simulink model "HANcoder_E407_GTSync_v5"  (R2018b)
settings: Solver=FixedStepDiscrete  StartTime=0.0  StopTime=1  FixedStep=0.01  RelTol=1e-3
PreLoadFcn:
  | librarySetup
  | eval([bdroot,'_startup']) %Calling [modelName]_startup.m
values from neighbouring files (symbols this model uses):
  basic_cycle_duration = TM_Reset_Board + COMP_duration    (= 170)    [HANcoder_E407_GTSync_v5_startup.m]
  comm_delay_estimation1 = round(comm_delay_measured*hardware_granularity/frequency_IRQ)    [HANcoder_E407_GTSync_v5_startup.m]
  comm_delay_estimation2 = round(comm_delay_measured*hardware_granularity/frequency_IRQ)    [HANcoder_E407_GTSync_v5_startup.m]
  COMM_Period = 25    [HANcoder_E407_GTSync_v5_startup.m]
  COMM_Phase1 = floor(COMM_Period/5)    [HANcoder_E407_GTSync_v5_startup.m]
  COMM_Phase2 = floor(4*COMM_Period/5)    [HANcoder_E407_GTSync_v5_startup.m]
  frequency_IRQ = 100    [HANcoder_E407_GTSync_v5_startup.m]
  HANtuneOverride = Simulink.Parameter    [HANcoder_E407_GTSync_v5_startup.m]
  idle_time_init = basic_cycle_duration*matrix_rows    (= 340)    [HANcoder_E407_GTSync_v5_startup.m]
  LED_ticks_toggle = 10000    [HANcoder_E407_GTSync_v5_startup.m]
  Master_Role = 1    [HANcoder_E407_GTSync_v5_startup.m]
  matrix_rows = 2    [HANcoder_E407_GTSync_v5_startup.m]
  MEX_Flag = 0    [HANcoder_E407_GTSync_v5_startup.m]
  Slave_Role = 2    [HANcoder_E407_GTSync_v5_startup.m]
  Sync_ID = 1    [HANcoder_E407_GTSync_v5_startup.m]
  TM_Check_Sync = TM_COMM_Sync   + COMM_duration    (= 30)    [HANcoder_E407_GTSync_v5_startup.m]
  TM_Check_TOuts = TM_Count_Vote3 + COMP_duration    (= 150)    [HANcoder_E407_GTSync_v5_startup.m]
  TM_Check_Vote1 = TM_COMM_Vote1  + COMM_duration    (= 70)    [HANcoder_E407_GTSync_v5_startup.m]
  TM_Check_Vote2 = TM_COMM_Vote2  + COMM_duration    (= 105)    [HANcoder_E407_GTSync_v5_startup.m]
  TM_Check_Vote3 = TM_COMM_Vote3  + COMM_duration    (= 140)    [HANcoder_E407_GTSync_v5_startup.m]
  TM_COMM_Sync = basic_cycle_start    (= 5)    [HANcoder_E407_GTSync_v5_startup.m]
  TM_COMM_Vote1 = TM_Vote_Dec    + COMP_duration    (= 45)    [HANcoder_E407_GTSync_v5_startup.m]
  TM_COMM_Vote2 = TM_Count_Vote1 + COMP_duration    (= 80)    [HANcoder_E407_GTSync_v5_startup.m]
  TM_COMM_Vote3 = TM_Count_Vote2 + COMP_duration    (= 115)    [HANcoder_E407_GTSync_v5_startup.m]
  TM_Count_Vote1 = TM_Check_Vote1 + COMP_duration    (= 75)    [HANcoder_E407_GTSync_v5_startup.m]
  TM_Count_Vote2 = TM_Check_Vote2 + COMP_duration    (= 110)    [HANcoder_E407_GTSync_v5_startup.m]
  TM_Count_Vote3 = TM_Check_Vote3 + COMP_duration    (= 145)    [HANcoder_E407_GTSync_v5_startup.m]
  TM_New_Master = TM_Check_TOuts + COMP_duration    (= 155)    [HANcoder_E407_GTSync_v5_startup.m]
  TM_Reset_Board = TM_Reset_Var   + COMP_duration    (= 165)    [HANcoder_E407_GTSync_v5_startup.m]
  TM_Reset_Var = TM_New_Master  + COMP_duration    (= 160)    [HANcoder_E407_GTSync_v5_startup.m]
  TM_Update_LT = TM_Check_Sync  + COMP_duration    (= 35)    [HANcoder_E407_GTSync_v5_startup.m]
  TM_Vote_Dec = TM_Update_LT   + COMP_duration    (= 40)    [HANcoder_E407_GTSync_v5_startup.m]
  Toggle_Flag = 1    [HANcoder_E407_GTSync_v5_startup.m]
  Vote1_ID = 12    [HANcoder_E407_GTSync_v5_startup.m]
  Vote2_ID = 22    [HANcoder_E407_GTSync_v5_startup.m]
  Vote3_ID = 32    [HANcoder_E407_GTSync_v5_startup.m]
undefined symbols (not defined in the file or in its folder): A0, A1, A2, A3, CON2
libraries: HANcoder_STM32_Target x25, hdlsllib x21, simulink x3, simulink_extras x1
(part 3 of 7)

== system HANcoder_E407_GTSync_v5/HANcoder STM32 Target - E407-STM32 algorithm/Global Ticks Increment/CAN Management/Initialization/RoleID and Global Time init ==
  note: Sync msg received!
  note: Reset variables
  note: Finish Initialization
  note: Role_ID Initialization
  Timeout Initialization : Inport
  Reference message received : Inport  Port=2
  Enable : EnablePort
  Constant : Constant  Priority=4  Value=Master_Role
  Constant1 : Constant  Priority=3  Value=Slave_Role
  Data Store Read : DataStoreRead  Priority=5  DataStoreName=Role_ID
  Data Store Write : DataStoreWrite  Priority=8  DataStoreName=Role_ID
  Data Store Write1 : DataStoreWrite  Priority=10  DataStoreName=sync_processed
  Data Store Write2 : DataStoreWrite  Priority=18  DataStoreName=Delay_Counter
  Data Store Write3 : DataStoreWrite  Priority=12  DataStoreName=New_Msg_Ready_CAN1
  Data Store Write4 : DataStoreWrite  Priority=16  DataStoreName=Initialization_Timeout
  Data Store Write5 : DataStoreWrite  Priority=14  DataStoreName=New_Msg_Ready_CAN2
  Global Time Initialization Master : Subsystem  Priority=2
  Global Time Initialization Slave : Subsystem  Priority=1
  RESET : Constant  Priority=15  Value=0  OutDataTypeStr=boolean
  RESET1 : Constant  Priority=17  Value=0  OutDataTypeStr=double
  RESET2 : Constant  Priority=11  Value=0  OutDataTypeStr=boolean
  RESET3 : Constant  Priority=13  Value=0  OutDataTypeStr=boolean
  SET : Constant  Priority=19
  "SET1 " : Constant  Priority=9  OutDataTypeStr=boolean
  Switch1 : Switch  Priority=6  Criteria=u2 > Threshold
  Switch2 : Switch  Priority=7  Criteria=u2 > Threshold
  Finish Initialization : Outport  OutputWhenDisabled=reset  InitialOutput=0
  wires:
  Switch1/1 -> Switch2/3
  Reference message received/1 -> Global Time Initialization Slave/Enable, Switch2/2
  Data Store Read/1 -> Switch1/3
  SET/1 -> Finish Initialization/1
  Constant/1 -> Switch1/1
  Constant1/1 -> Switch2/1
  Switch2/1 -> Data Store Write/1
  RESET/1 -> Data Store Write4/1
  Timeout Initialization/1 -> Switch1/2, Global Time Initialization Master/Enable
  RESET1/1 -> Data Store Write2/1
  "SET1 "/1 -> Data Store Write1/1
  RESET2/1 -> Data Store Write3/1
  RESET3/1 -> Data Store Write5/1

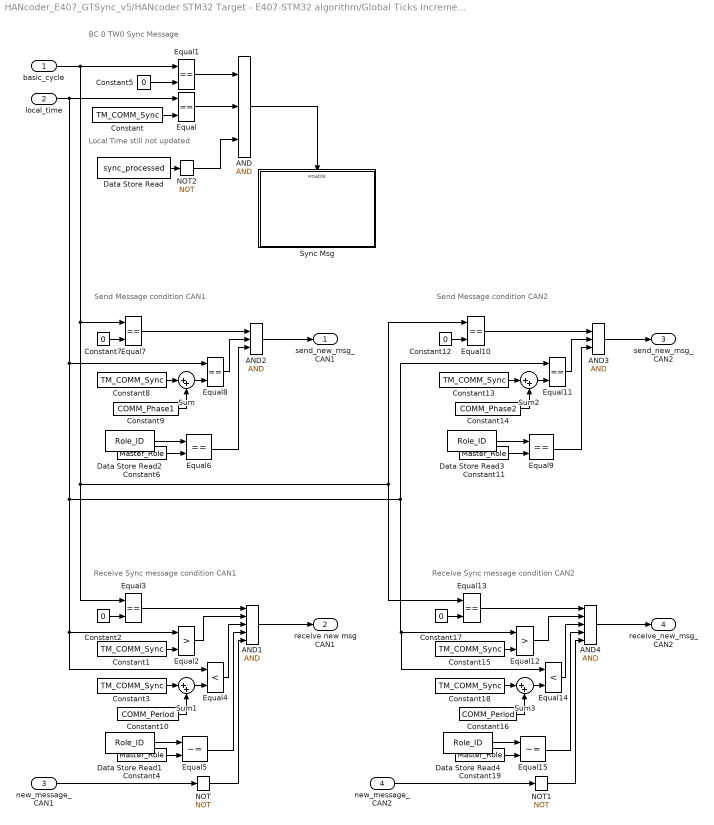
== system HANcoder_E407_GTSync_v5/HANcoder STM32 Target - E407-STM32 algorithm/Global Ticks Increment/CAN Management/Matrix Cycle Manager/COMM Task - Sync BC0 ==
  note: BC 0 TW0
      | Sync Message
  note: Receive Sync message condition CAN1
  note: Send Message condition CAN1
  note: Send Message condition CAN2
  note: Receive Sync message condition CAN2
  note: Local Time still not updated
  basic_cycle : Inport
  local_time : Inport  Port=2
  new_message_CAN1 : Inport  Port=3
  new_message_CAN2 : Inport  Port=4
  AND : Logic  Inputs=3  IconShape=distinctive  AllPortsSameDT=off  OutDataTypeStr=boolean
  AND1 : Logic  Inputs=5  IconShape=distinctive  AllPortsSameDT=off  OutDataTypeStr=boolean
  AND2 : Logic  Inputs=3  IconShape=distinctive  AllPortsSameDT=off  OutDataTypeStr=boolean
  AND3 : Logic  Inputs=3  IconShape=distinctive  AllPortsSameDT=off  OutDataTypeStr=boolean
  AND4 : Logic  Inputs=5  IconShape=distinctive  AllPortsSameDT=off  OutDataTypeStr=boolean
  Constant{,1,3,8,13,15,18} (7 alike) : Constant  Value=TM_COMM_Sync
  Constant10 : Constant  Value=COMM_Period
  Constant{4,6,11,19} (4 alike) : Constant  Value=Master_Role
  Constant12 : Constant  Value=0
  Constant14 : Constant  Value=COMM_Phase2
  Constant16 : Constant  Value=COMM_Period
  Constant17 : Constant  Value=0  OutDataTypeStr=uint8
  Constant2 : Constant  Value=0  OutDataTypeStr=uint8
  Constant5 : Constant  Value=0
  Constant7 : Constant  Value=0
  Constant9 : Constant  Value=COMM_Phase1
  Data Store Read : DataStoreRead  DataStoreName=sync_processed
  Data Store Read{1..4} (4 alike) : DataStoreRead  DataStoreName=Role_ID
  Equal{,1,3,6..11,13} (10 alike) : RelationalOperator  Operator===  OutDataTypeStr=boolean  RndMeth=Simplest
  Equal12 : RelationalOperator  Operator=>  OutDataTypeStr=boolean  RndMeth=Simplest
  Equal14 : RelationalOperator  Operator=<  OutDataTypeStr=boolean  RndMeth=Simplest
  Equal15 : RelationalOperator  Operator=~=  OutDataTypeStr=boolean  RndMeth=Simplest
  Equal2 : RelationalOperator  Operator=>  OutDataTypeStr=boolean  RndMeth=Simplest
  Equal4 : RelationalOperator  Operator=<  OutDataTypeStr=boolean  RndMeth=Simplest
  Equal5 : RelationalOperator  Operator=~=  OutDataTypeStr=boolean  RndMeth=Simplest
  NOT : Logic  Operator=NOT  IconShape=distinctive  AllPortsSameDT=off  OutDataTypeStr=boolean
  NOT1 : Logic  Operator=NOT  IconShape=distinctive  AllPortsSameDT=off  OutDataTypeStr=boolean
  NOT2 : Logic  Operator=NOT  IconShape=distinctive  AllPortsSameDT=off  OutDataTypeStr=boolean
  Sum{,1..3} (4 alike) : Sum  Inputs=|++
  Sync Msg : Subsystem  Priority=20
  send_new_msg_CAN1 : Outport
  receive new msg CAN1 : Outport  Port=2
  send_new_msg_CAN2 : Outport  Port=3
  receive_new_msg_CAN2 : Outport  Port=4
  wires:
  Constant/1 -> Equal/2
  Constant5/1 -> Equal1/2
  Equal1/1 -> AND/1
  Equal/1 -> AND/2
  AND/1 -> Sync Msg/Enable
  Data Store Read1/1 -> Equal5/1
  Constant4/1 -> Equal5/2
  AND1/1 -> receive new msg CAN1/1
  Equal2/1 -> AND1/2
  Equal5/1 -> AND1/4
  Equal3/1 -> AND1/1
  Equal4/1 -> AND1/3
  Constant3/1 -> Sum1/1
  Constant1/1 -> Equal2/2
  Constant2/1 -> Equal3/2
  Constant6/1 -> Equal6/2
  Data Store Read2/1 -> Equal6/1
  Constant7/1 -> Equal7/2
  Equal7/1 -> AND2/1
  AND2/1 -> send_new_msg_CAN1/1
  Equal8/1 -> AND2/2
  Equal6/1 -> AND2/3
  Constant8/1 -> Sum/1
  Sum/1 -> Equal8/2
  Constant9/1 -> Sum/2
  Constant10/1 -> Sum1/2
  Sum1/1 -> Equal4/2
  new_message_CAN1/1 -> NOT/1
  NOT/1 -> AND1/5
  Constant14/1 -> Sum2/2
  Sum2/1 -> Equal11/2
  Constant13/1 -> Sum2/1
  Equal9/1 -> AND3/3
  Equal11/1 -> AND3/2
  AND3/1 -> send_new_msg_CAN2/1
  Equal10/1 -> AND3/1
  Constant12/1 -> Equal10/2
  Data Store Read3/1 -> Equal9/1
  Constant11/1 -> Equal9/2
  local_time/1 -> Equal14/1, Equal12/1, Equal11/1, Equal4/1, Equal2/1, Equal8/1, Equal/1
  basic_cycle/1 -> Equal7/1, Equal10/1, Equal13/1, Equal3/1, Equal1/1
  NOT1/1 -> AND4/5
  new_message_CAN2/1 -> NOT1/1
  Sum3/1 -> Equal14/2
  Constant16/1 -> Sum3/2
  Constant17/1 -> Equal13/2
  Constant15/1 -> Equal12/2
  Constant18/1 -> Sum3/1
  Equal14/1 -> AND4/3
  Equal13/1 -> AND4/1
  Equal15/1 -> AND4/4
  Equal12/1 -> AND4/2
  AND4/1 -> receive_new_msg_CAN2/1
  Constant19/1 -> Equal15/2
  Data Store Read4/1 -> Equal15/1
  Data Store Read/1 -> NOT2/1
  NOT2/1 -> AND/3

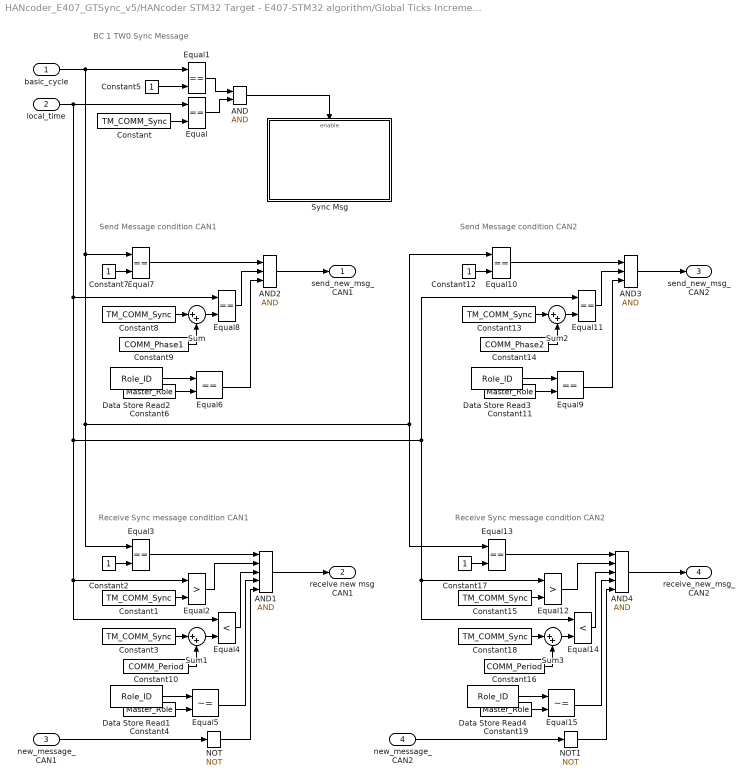
== system HANcoder_E407_GTSync_v5/HANcoder STM32 Target - E407-STM32 algorithm/Global Ticks Increment/CAN Management/Matrix Cycle Manager/COMM Task - Sync BC1 ==
  note: BC 1 TW0
      | Sync Message
  note: Receive Sync message condition CAN1
  note: Send Message condition CAN1
  note: Send Message condition CAN2
  note: Receive Sync message condition CAN2
  basic_cycle : Inport
  local_time : Inport  Port=2
  new_message_CAN1 : Inport  Port=3
  new_message_CAN2 : Inport  Port=4
  AND : Logic  IconShape=distinctive  AllPortsSameDT=off  OutDataTypeStr=boolean
  AND1 : Logic  Inputs=5  IconShape=distinctive  AllPortsSameDT=off  OutDataTypeStr=boolean
  AND2 : Logic  Inputs=3  IconShape=distinctive  AllPortsSameDT=off  OutDataTypeStr=boolean
  AND3 : Logic  Inputs=3  IconShape=distinctive  AllPortsSameDT=off  OutDataTypeStr=boolean
  AND4 : Logic  Inputs=5  IconShape=distinctive  AllPortsSameDT=off  OutDataTypeStr=boolean
  Constant{,1,3,8,13,15,18} (7 alike) : Constant  Value=TM_COMM_Sync
  Constant10 : Constant  Value=COMM_Period
  Constant{4,6,11,19} (4 alike) : Constant  Value=Master_Role
  Constant12 : Constant
  Constant14 : Constant  Value=COMM_Phase2
  Constant16 : Constant  Value=COMM_Period
  Constant17 : Constant  OutDataTypeStr=uint8
  Constant2 : Constant  OutDataTypeStr=uint8
  Constant5 : Constant
  Constant7 : Constant
  Constant9 : Constant  Value=COMM_Phase1
  Data Store Read{1..4} (4 alike) : DataStoreRead  DataStoreName=Role_ID
  Equal{,1,3,6..11,13} (10 alike) : RelationalOperator  Operator===  OutDataTypeStr=boolean  RndMeth=Simplest
  Equal12 : RelationalOperator  Operator=>  OutDataTypeStr=boolean  RndMeth=Simplest
  Equal14 : RelationalOperator  Operator=<  OutDataTypeStr=boolean  RndMeth=Simplest
  Equal15 : RelationalOperator  Operator=~=  OutDataTypeStr=boolean  RndMeth=Simplest
  Equal2 : RelationalOperator  Operator=>  OutDataTypeStr=boolean  RndMeth=Simplest
  Equal4 : RelationalOperator  Operator=<  OutDataTypeStr=boolean  RndMeth=Simplest
  Equal5 : RelationalOperator  Operator=~=  OutDataTypeStr=boolean  RndMeth=Simplest
  NOT : Logic  Operator=NOT  IconShape=distinctive  AllPortsSameDT=off  OutDataTypeStr=boolean
  NOT1 : Logic  Operator=NOT  IconShape=distinctive  AllPortsSameDT=off  OutDataTypeStr=boolean
  Sum{,1..3} (4 alike) : Sum  Inputs=|++
  Sync Msg : Subsystem
  send_new_msg_CAN1 : Outport
  receive new msg CAN1 : Outport  Port=2
  send_new_msg_CAN2 : Outport  Port=3
  receive_new_msg_CAN2 : Outport  Port=4
  wires:
  Constant/1 -> Equal/2
  Constant5/1 -> Equal1/2
  Equal1/1 -> AND/1
  Equal/1 -> AND/2
  AND/1 -> Sync Msg/Enable
  Data Store Read1/1 -> Equal5/1
  Constant4/1 -> Equal5/2
  AND1/1 -> receive new msg CAN1/1
  Equal2/1 -> AND1/2
  Equal5/1 -> AND1/4
  Equal3/1 -> AND1/1
  Equal4/1 -> AND1/3
  Constant3/1 -> Sum1/1
  Constant1/1 -> Equal2/2
  Constant2/1 -> Equal3/2
  Constant6/1 -> Equal6/2
  Data Store Read2/1 -> Equal6/1
  Constant7/1 -> Equal7/2
  Equal7/1 -> AND2/1
  AND2/1 -> send_new_msg_CAN1/1
  Equal8/1 -> AND2/2
  Equal6/1 -> AND2/3
  Constant8/1 -> Sum/1
  Sum/1 -> Equal8/2
  Constant9/1 -> Sum/2
  Constant10/1 -> Sum1/2
  Sum1/1 -> Equal4/2
  new_message_CAN1/1 -> NOT/1
  NOT/1 -> AND1/5
  Constant14/1 -> Sum2/2
  Sum2/1 -> Equal11/2
  Constant13/1 -> Sum2/1
  Equal9/1 -> AND3/3
  Equal11/1 -> AND3/2
  AND3/1 -> send_new_msg_CAN2/1
  Equal10/1 -> AND3/1
  Constant12/1 -> Equal10/2
  Data Store Read3/1 -> Equal9/1
  Constant11/1 -> Equal9/2
  local_time/1 -> Equal14/1, Equal12/1, Equal11/1, Equal4/1, Equal2/1, Equal8/1, Equal/1
  basic_cycle/1 -> Equal7/1, Equal10/1, Equal13/1, Equal3/1, Equal1/1
  NOT1/1 -> AND4/5
  new_message_CAN2/1 -> NOT1/1
  Sum3/1 -> Equal14/2
  Constant16/1 -> Sum3/2
  Constant17/1 -> Equal13/2
  Constant15/1 -> Equal12/2
  Constant18/1 -> Sum3/1
  Equal14/1 -> AND4/3
  Equal13/1 -> AND4/1
  Equal15/1 -> AND4/4
  Equal12/1 -> AND4/2
  AND4/1 -> receive_new_msg_CAN2/1
  Constant19/1 -> Equal15/2
  Data Store Read4/1 -> Equal15/1

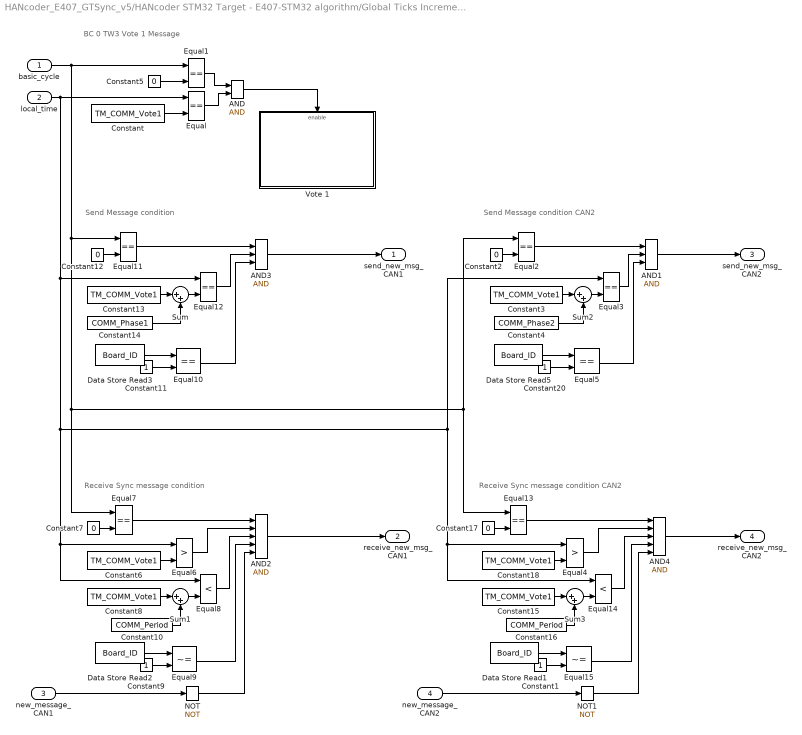
== system HANcoder_E407_GTSync_v5/HANcoder STM32 Target - E407-STM32 algorithm/Global Ticks Increment/CAN Management/Matrix Cycle Manager/COMM Task - Vote1 ==
  note: BC 0 TW3
      | Vote 1 Message
  note: Send Message condition
  note: Receive Sync message condition
  note: Send Message condition CAN2
  note: Receive Sync message condition CAN2
  basic_cycle : Inport
  local_time : Inport  Port=2
  new_message_CAN1 : Inport  Port=3
  new_message_CAN2 : Inport  Port=4
  AND : Logic  IconShape=distinctive  AllPortsSameDT=off  OutDataTypeStr=boolean
  AND1 : Logic  Inputs=3  IconShape=distinctive  AllPortsSameDT=off  OutDataTypeStr=boolean
  AND2 : Logic  Inputs=5  IconShape=distinctive  AllPortsSameDT=off  OutDataTypeStr=boolean
  AND3 : Logic  Inputs=3  IconShape=distinctive  AllPortsSameDT=off  OutDataTypeStr=boolean
  AND4 : Logic  Inputs=5  IconShape=distinctive  AllPortsSameDT=off  OutDataTypeStr=boolean
  Constant{,3,6,8,13,15,18} (7 alike) : Constant  Value=TM_COMM_Vote1
  Constant{1,9,11,20} (4 alike) : Constant
  Constant10 : Constant  Value=COMM_Period
  Constant12 : Constant  Value=0
  Constant14 : Constant  Value=COMM_Phase1
  Constant16 : Constant  Value=COMM_Period
  Constant17 : Constant  Value=0  OutDataTypeStr=uint8
  Constant2 : Constant  Value=0
  Constant4 : Constant  Value=COMM_Phase2
  Constant5 : Constant  Value=0
  Constant7 : Constant  Value=0  OutDataTypeStr=uint8
  Data Store Read{1..3,5} (4 alike) : DataStoreRead  DataStoreName=Board_ID
  Equal{,1..3,5,7,10..13} (10 alike) : RelationalOperator  Operator===  OutDataTypeStr=boolean  RndMeth=Simplest
  Equal14 : RelationalOperator  Operator=<  OutDataTypeStr=boolean  RndMeth=Simplest
  Equal15 : RelationalOperator  Operator=~=  OutDataTypeStr=boolean  RndMeth=Simplest
  Equal4 : RelationalOperator  Operator=>  OutDataTypeStr=boolean  RndMeth=Simplest
  Equal6 : RelationalOperator  Operator=>  OutDataTypeStr=boolean  RndMeth=Simplest
  Equal8 : RelationalOperator  Operator=<  OutDataTypeStr=boolean  RndMeth=Simplest
  Equal9 : RelationalOperator  Operator=~=  OutDataTypeStr=boolean  RndMeth=Simplest
  NOT : Logic  Operator=NOT  IconShape=distinctive  AllPortsSameDT=off  OutDataTypeStr=boolean
  NOT1 : Logic  Operator=NOT  IconShape=distinctive  AllPortsSameDT=off  OutDataTypeStr=boolean
  Sum{,1..3} (4 alike) : Sum  Inputs=|++
  Vote 1 : Subsystem  Priority=20
  send_new_msg_CAN1 : Outport
  receive_new_msg_CAN1 : Outport  Port=2
  send_new_msg_CAN2 : Outport  Port=3
  receive_new_msg_CAN2 : Outport  Port=4
  wires:
  AND/1 -> Vote 1/Enable
  Equal/1 -> AND/2
  Equal1/1 -> AND/1
  Constant5/1 -> Equal1/2
  Constant/1 -> Equal/2
  Constant11/1 -> Equal10/2
  Sum/1 -> Equal12/2
  Constant13/1 -> Sum/1
  Constant6/1 -> Equal6/2
  Constant7/1 -> Equal7/2
  Constant9/1 -> Equal9/2
  Equal9/1 -> AND2/4
  Data Store Read2/1 -> Equal9/1
  Equal8/1 -> AND2/3
  Equal7/1 -> AND2/1
  Equal6/1 -> AND2/2
  Equal12/1 -> AND3/2
  Data Store Read3/1 -> Equal10/1
  Constant10/1 -> Sum1/2
  Constant8/1 -> Sum1/1
  Equal10/1 -> AND3/3
  Sum1/1 -> Equal8/2
  Constant12/1 -> Equal11/2
  Constant14/1 -> Sum/2
  Equal11/1 -> AND3/1
  new_message_CAN1/1 -> NOT/1
  NOT/1 -> AND2/5
  AND3/1 -> send_new_msg_CAN1/1
  AND2/1 -> receive_new_msg_CAN1/1
  Data Store Read5/1 -> Equal5/1
  Equal2/1 -> AND1/1
  Equal3/1 -> AND1/2
  AND1/1 -> send_new_msg_CAN2/1
  Constant2/1 -> Equal2/2
  Sum2/1 -> Equal3/2
  Constant3/1 -> Sum2/1
  Equal5/1 -> AND1/3
  Constant20/1 -> Equal5/2
  Constant4/1 -> Sum2/2
  local_time/1 -> Equal12/1, Equal4/1, Equal14/1, Equal3/1, Equal6/1, Equal8/1, Equal/1
  Constant17/1 -> Equal13/2
  AND4/1 -> receive_new_msg_CAN2/1
  Constant15/1 -> Sum3/1
  basic_cycle/1 -> Equal11/1, Equal13/1, Equal2/1, Equal7/1, Equal1/1
  Equal14/1 -> AND4/3
  Constant18/1 -> Equal4/2
  Constant1/1 -> Equal15/2
  Equal15/1 -> AND4/4
  Equal13/1 -> AND4/1
  NOT1/1 -> AND4/5
  Constant16/1 -> Sum3/2
  Sum3/1 -> Equal14/2
  Equal4/1 -> AND4/2
  Data Store Read1/1 -> Equal15/1
  new_message_CAN2/1 -> NOT1/1

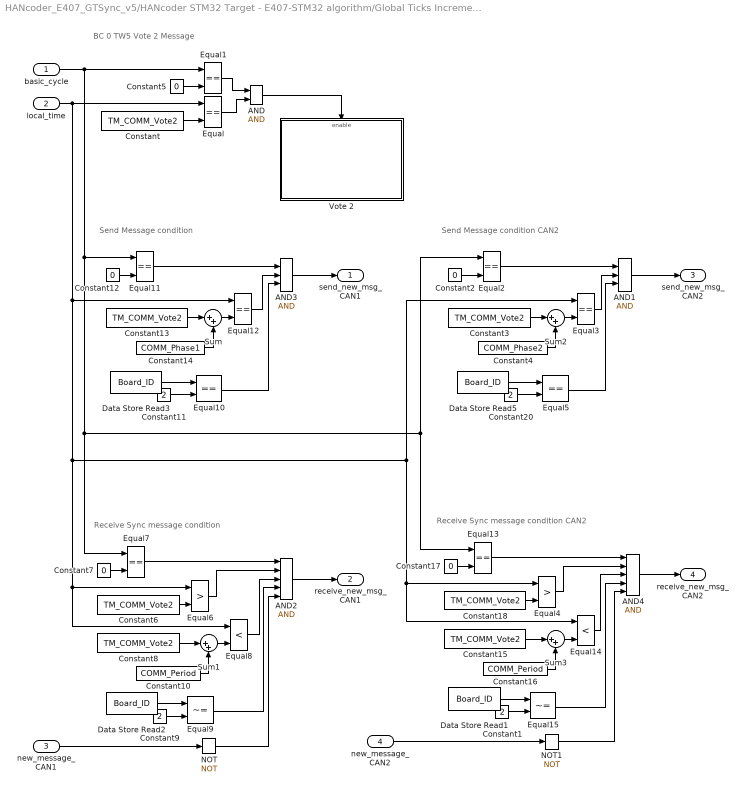
== system HANcoder_E407_GTSync_v5/HANcoder STM32 Target - E407-STM32 algorithm/Global Ticks Increment/CAN Management/Matrix Cycle Manager/COMM Task - Vote2 ==
  note: BC 0 TW5
      | Vote 2 Message
  note: Receive Sync message condition
  note: Send Message condition
  note: Receive Sync message condition CAN2
  note: Send Message condition CAN2
  basic_cycle : Inport
  local_time : Inport  Port=2
  new_message_CAN1 : Inport  Port=3
  new_message_CAN2 : Inport  Port=4
  AND : Logic  IconShape=distinctive  AllPortsSameDT=off  OutDataTypeStr=boolean
  AND1 : Logic  Inputs=3  IconShape=distinctive  AllPortsSameDT=off  OutDataTypeStr=boolean
  AND2 : Logic  Inputs=5  IconShape=distinctive  AllPortsSameDT=off  OutDataTypeStr=boolean
  AND3 : Logic  Inputs=3  IconShape=distinctive  AllPortsSameDT=off  OutDataTypeStr=boolean
  AND4 : Logic  Inputs=5  IconShape=distinctive  AllPortsSameDT=off  OutDataTypeStr=boolean
  Constant{,3,6,8,13,15,18} (7 alike) : Constant  Value=TM_COMM_Vote2
  Constant{1,9,11,20} (4 alike) : Constant  Value=2
  Constant10 : Constant  Value=COMM_Period
  Constant12 : Constant  Value=0
  Constant14 : Constant  Value=COMM_Phase1
  Constant16 : Constant  Value=COMM_Period
  Constant17 : Constant  Value=0  OutDataTypeStr=uint8
  Constant2 : Constant  Value=0
  Constant4 : Constant  Value=COMM_Phase2
  Constant5 : Constant  Value=0
  Constant7 : Constant  Value=0  OutDataTypeStr=uint8
  Data Store Read{1..3,5} (4 alike) : DataStoreRead  DataStoreName=Board_ID
  Equal{,1..3,5,7,10..13} (10 alike) : RelationalOperator  Operator===  OutDataTypeStr=boolean  RndMeth=Simplest
  Equal14 : RelationalOperator  Operator=<  OutDataTypeStr=boolean  RndMeth=Simplest
  Equal15 : RelationalOperator  Operator=~=  OutDataTypeStr=boolean  RndMeth=Simplest
  Equal4 : RelationalOperator  Operator=>  OutDataTypeStr=boolean  RndMeth=Simplest
  Equal6 : RelationalOperator  Operator=>  OutDataTypeStr=boolean  RndMeth=Simplest
  Equal8 : RelationalOperator  Operator=<  OutDataTypeStr=boolean  RndMeth=Simplest
  Equal9 : RelationalOperator  Operator=~=  OutDataTypeStr=boolean  RndMeth=Simplest
  NOT : Logic  Operator=NOT  IconShape=distinctive  AllPortsSameDT=off  OutDataTypeStr=boolean
  NOT1 : Logic  Operator=NOT  IconShape=distinctive  AllPortsSameDT=off  OutDataTypeStr=boolean
  Sum{,1..3} (4 alike) : Sum  Inputs=|++
  Vote 2 : Subsystem
  send_new_msg_CAN1 : Outport
  receive_new_msg_CAN1 : Outport  Port=2
  send_new_msg_CAN2 : Outport  Port=3
  receive_new_msg_CAN2 : Outport  Port=4
  wires:
  Constant/1 -> Equal/2
  Constant5/1 -> Equal1/2
  Equal1/1 -> AND/1
  Equal/1 -> AND/2
  AND/1 -> Vote 2/Enable
  Constant12/1 -> Equal11/2
  Equal11/1 -> AND3/1
  Constant14/1 -> Sum/2
  Constant10/1 -> Sum1/2
  Equal10/1 -> AND3/3
  Sum1/1 -> Equal8/2
  Constant8/1 -> Sum1/1
  Data Store Read3/1 -> Equal10/1
  Equal12/1 -> AND3/2
  Equal6/1 -> AND2/2
  Equal8/1 -> AND2/3
  Data Store Read2/1 -> Equal9/1
  Equal9/1 -> AND2/4
  Constant7/1 -> Equal7/2
  Equal7/1 -> AND2/1
  Constant13/1 -> Sum/1
  Constant11/1 -> Equal10/2
  Sum/1 -> Equal12/2
  Constant6/1 -> Equal6/2
  Constant9/1 -> Equal9/2
  new_message_CAN1/1 -> NOT/1
  NOT/1 -> AND2/5
  AND3/1 -> send_new_msg_CAN1/1
  AND2/1 -> receive_new_msg_CAN1/1
  Constant2/1 -> Equal2/2
  AND1/1 -> send_new_msg_CAN2/1
  Equal2/1 -> AND1/1
  new_message_CAN2/1 -> NOT1/1
  Data Store Read5/1 -> Equal5/1
  Constant1/1 -> Equal15/2
  local_time/1 -> Equal12/1, Equal3/1, Equal4/1, Equal14/1, Equal6/1, Equal8/1, Equal/1
  Equal13/1 -> AND4/1
  Equal15/1 -> AND4/4
  Equal14/1 -> AND4/3
  Constant15/1 -> Sum3/1
  Constant18/1 -> Equal4/2
  Constant3/1 -> Sum2/1
  Constant17/1 -> Equal13/2
  Equal3/1 -> AND1/2
  AND4/1 -> receive_new_msg_CAN2/1
  Constant20/1 -> Equal5/2
  Constant4/1 -> Sum2/2
  Equal4/1 -> AND4/2
  NOT1/1 -> AND4/5
  Constant16/1 -> Sum3/2
  Sum3/1 -> Equal14/2
  Sum2/1 -> Equal3/2
  Data Store Read1/1 -> Equal15/1
  basic_cycle/1 -> Equal11/1, Equal13/1, Equal2/1, Equal7/1, Equal1/1
  Equal5/1 -> AND1/3

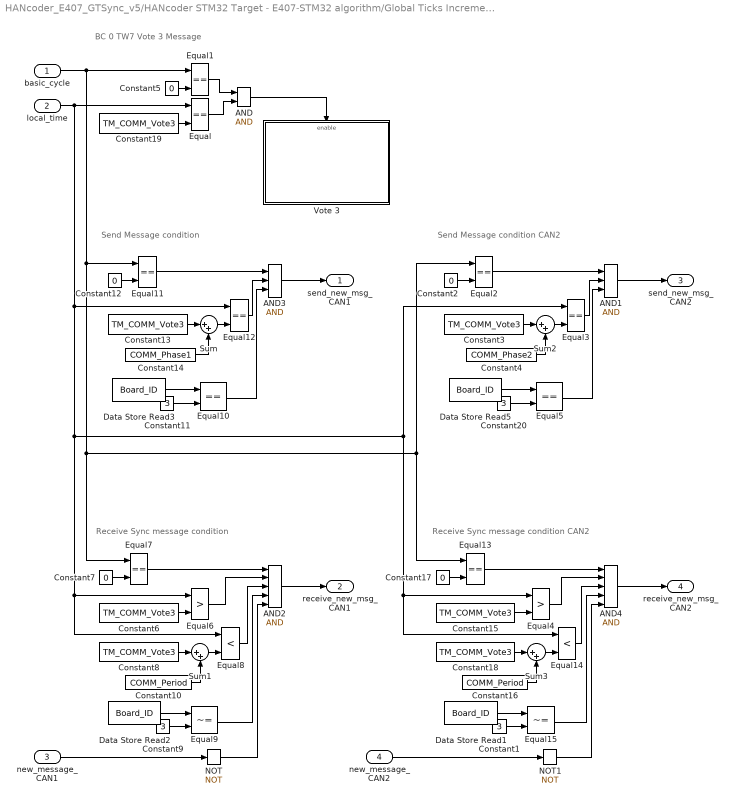
== system HANcoder_E407_GTSync_v5/HANcoder STM32 Target - E407-STM32 algorithm/Global Ticks Increment/CAN Management/Matrix Cycle Manager/COMM Task - Vote3 ==
  note: BC 0 TW7
      | Vote 3 Message
  note: Receive Sync message condition
  note: Send Message condition
  note: Receive Sync message condition CAN2
  note: Send Message condition CAN2
  basic_cycle : Inport
  local_time : Inport  Port=2
  new_message_CAN1 : Inport  Port=3
  new_message_CAN2 : Inport  Port=4
  AND : Logic  IconShape=distinctive  AllPortsSameDT=off  OutDataTypeStr=boolean
  AND1 : Logic  Inputs=3  IconShape=distinctive  AllPortsSameDT=off  OutDataTypeStr=boolean
  AND2 : Logic  Inputs=5  IconShape=distinctive  AllPortsSameDT=off  OutDataTypeStr=boolean
  AND3 : Logic  Inputs=3  IconShape=distinctive  AllPortsSameDT=off  OutDataTypeStr=boolean
  AND4 : Logic  Inputs=5  IconShape=distinctive  AllPortsSameDT=off  OutDataTypeStr=boolean
  Constant{1,9,11,20} (4 alike) : Constant  Value=3
  Constant10 : Constant  Value=COMM_Period
  Constant12 : Constant  Value=0
  Constant{3,6,8,13,15,18..19} (7 alike) : Constant  Value=TM_COMM_Vote3
  Constant14 : Constant  Value=COMM_Phase1
  Constant16 : Constant  Value=COMM_Period
  Constant17 : Constant  Value=0  OutDataTypeStr=uint8
  Constant2 : Constant  Value=0
  Constant4 : Constant  Value=COMM_Phase2
  Constant5 : Constant  Value=0
  Constant7 : Constant  Value=0  OutDataTypeStr=uint8
  Data Store Read{1..3,5} (4 alike) : DataStoreRead  DataStoreName=Board_ID
  Equal{,1..3,5,7,10..13} (10 alike) : RelationalOperator  Operator===  OutDataTypeStr=boolean  RndMeth=Simplest
  Equal14 : RelationalOperator  Operator=<  OutDataTypeStr=boolean  RndMeth=Simplest
  Equal15 : RelationalOperator  Operator=~=  OutDataTypeStr=boolean  RndMeth=Simplest
  Equal4 : RelationalOperator  Operator=>  OutDataTypeStr=boolean  RndMeth=Simplest
  Equal6 : RelationalOperator  Operator=>  OutDataTypeStr=boolean  RndMeth=Simplest
  Equal8 : RelationalOperator  Operator=<  OutDataTypeStr=boolean  RndMeth=Simplest
  Equal9 : RelationalOperator  Operator=~=  OutDataTypeStr=boolean  RndMeth=Simplest
  NOT : Logic  Operator=NOT  IconShape=distinctive  AllPortsSameDT=off  OutDataTypeStr=boolean
  NOT1 : Logic  Operator=NOT  IconShape=distinctive  AllPortsSameDT=off  OutDataTypeStr=boolean
  Sum{,1..3} (4 alike) : Sum  Inputs=|++
  Vote 3 : Subsystem
  send_new_msg_CAN1 : Outport
  receive_new_msg_CAN1 : Outport  Port=2
  send_new_msg_CAN2 : Outport  Port=3
  receive_new_msg_CAN2 : Outport  Port=4
  wires:
  AND/1 -> Vote 3/Enable
  Equal/1 -> AND/2
  Equal1/1 -> AND/1
  Constant5/1 -> Equal1/2
  Constant19/1 -> Equal/2
  AND2/1 -> receive_new_msg_CAN1/1
  Constant12/1 -> Equal11/2
  Equal11/1 -> AND3/1
  Constant14/1 -> Sum/2
  Constant10/1 -> Sum1/2
  Equal10/1 -> AND3/3
  Sum1/1 -> Equal8/2
  Constant8/1 -> Sum1/1
  Data Store Read3/1 -> Equal10/1
  Equal12/1 -> AND3/2
  Equal6/1 -> AND2/2
  Equal8/1 -> AND2/3
  Data Store Read2/1 -> Equal9/1
  Equal9/1 -> AND2/4
  Constant7/1 -> Equal7/2
  Equal7/1 -> AND2/1
  Constant13/1 -> Sum/1
  Constant11/1 -> Equal10/2
  Sum/1 -> Equal12/2
  Constant6/1 -> Equal6/2
  Constant9/1 -> Equal9/2
  new_message_CAN1/1 -> NOT/1
  NOT/1 -> AND2/5
  AND3/1 -> send_new_msg_CAN1/1
  Constant16/1 -> Sum3/2
  Sum3/1 -> Equal14/2
  Equal4/1 -> AND4/2
  Equal5/1 -> AND1/3
  NOT1/1 -> AND4/5
  Constant17/1 -> Equal13/2
  Data Store Read1/1 -> Equal15/1
  Constant3/1 -> Sum2/1
  Constant4/1 -> Sum2/2
  Equal3/1 -> AND1/2
  Constant20/1 -> Equal5/2
  AND4/1 -> receive_new_msg_CAN2/1
  Equal14/1 -> AND4/3
  Constant18/1 -> Sum3/1
  Constant15/1 -> Equal4/2
  Constant1/1 -> Equal15/2
  Equal13/1 -> AND4/1
  Data Store Read5/1 -> Equal5/1
  Equal15/1 -> AND4/4
  Sum2/1 -> Equal3/2
  Constant2/1 -> Equal2/2
  Equal2/1 -> AND1/1
  new_message_CAN2/1 -> NOT1/1
  basic_cycle/1 -> Equal11/1, Equal2/1, Equal13/1, Equal7/1, Equal1/1
  AND1/1 -> send_new_msg_CAN2/1
  local_time/1 -> Equal12/1, Equal6/1, Equal8/1, Equal4/1, Equal14/1, Equal3/1, Equal/1

== system HANcoder_E407_GTSync_v5/HANcoder STM32 Target - E407-STM32 algorithm/Global Ticks Increment/CAN Management/Matrix Cycle Manager/COMP Task - Check Timeouts ==
  note: BC 0 TW9
      | Timeout check
  basic cycle : Inport
  local time : Inport  Port=2
  AND : Logic  IconShape=distinctive  AllPortsSameDT=off  OutDataTypeStr=boolean
  Constant : Constant  Value=TM_Check_TOuts
  Constant5 : Constant  Value=0
  Equal : RelationalOperator  Operator===  OutDataTypeStr=boolean  RndMeth=Simplest
  Equal1 : RelationalOperator  Operator===  OutDataTypeStr=boolean  RndMeth=Simplest
  Timeout and Board error counter : Subsystem
  wires:
  Constant/1 -> Equal/2
  local time/1 -> Equal/1
  Constant5/1 -> Equal1/2
  basic cycle/1 -> Equal1/1
  Equal1/1 -> AND/1
  Equal/1 -> AND/2
  AND/1 -> Timeout and Board error counter/Enable

== system HANcoder_E407_GTSync_v5/HANcoder STM32 Target - E407-STM32 algorithm/Global Ticks Increment/CAN Management/Matrix Cycle Manager/COMP Task - New Master ==
  note: BC 0 TW10
      | New Master decision
  basic cycle : Inport
  local time : Inport  Port=2
  AND : Logic  IconShape=distinctive  AllPortsSameDT=off  OutDataTypeStr=boolean
  Constant : Constant  Value=TM_New_Master
  Constant5 : Constant  Value=0
  Equal : RelationalOperator  Operator===  OutDataTypeStr=boolean  RndMeth=Simplest
  Equal1 : RelationalOperator  Operator===  OutDataTypeStr=boolean  RndMeth=Simplest
  New Master : Subsystem
  wires:
  AND/1 -> New Master/Enable
  Equal/1 -> AND/2
  Equal1/1 -> AND/1
  basic cycle/1 -> Equal1/1
  Constant5/1 -> Equal1/2
  local time/1 -> Equal/1
  Constant/1 -> Equal/2

== system HANcoder_E407_GTSync_v5/HANcoder STM32 Target - E407-STM32 algorithm/Global Ticks Increment/CAN Management/Matrix Cycle Manager/COMP Task - Reset Board ==
  note: BC 0 TW12
      | Reset Board
  basic cycle : Inport
  local time : Inport  Port=2
  AND : Logic  Inputs=3  IconShape=distinctive  AllPortsSameDT=off  OutDataTypeStr=boolean
  Constant : Constant  Value=TM_Reset_Board
  Constant5 : Constant  Value=0
  Data Store Read : DataStoreRead  DataStoreName=Reset_Board
  Equal : RelationalOperator  Operator===  OutDataTypeStr=boolean  RndMeth=Simplest
  Equal1 : RelationalOperator  Operator===  OutDataTypeStr=boolean  RndMeth=Simplest
  RESET Board - Return to initialization : Subsystem  TreatAsAtomicUnit=on
  wires:
  AND/1 -> RESET Board - Return to initialization/Enable
  Equal/1 -> AND/2
  Equal1/1 -> AND/1
  basic cycle/1 -> Equal1/1
  Constant5/1 -> Equal1/2
  local time/1 -> Equal/1
  Constant/1 -> Equal/2
  Data Store Read/1 -> AND/3  "reset_s"

== system HANcoder_E407_GTSync_v5/HANcoder STM32 Target - E407-STM32 algorithm/Global Ticks Increment/CAN Management/Matrix Cycle Manager/COMP Task - Reset Variables BC0 ==
  note: BC 0 TW11
      | Reset variables
  basic cycle : Inport
  local time : Inport  Port=2
  AND : Logic  IconShape=distinctive  AllPortsSameDT=off  OutDataTypeStr=boolean
  Constant : Constant  Value=TM_Reset_Var
  Constant5 : Constant  Value=0
  Equal : RelationalOperator  Operator===  OutDataTypeStr=boolean  RndMeth=Simplest
  Equal1 : RelationalOperator  Operator===  OutDataTypeStr=boolean  RndMeth=Simplest
  Reset variables : Subsystem
  wires:
  Constant/1 -> Equal/2
  local time/1 -> Equal/1
  Constant5/1 -> Equal1/2
  basic cycle/1 -> Equal1/1
  Equal1/1 -> AND/1
  Equal/1 -> AND/2
  AND/1 -> Reset variables/Enable

== system HANcoder_E407_GTSync_v5/HANcoder STM32 Target - E407-STM32 algorithm/Global Ticks Increment/CAN Management/Matrix Cycle Manager/COMP Task - Reset Variables BC1 ==
  note: BC 1 TW11
      | Reset Variables
  basic cycle : Inport
  local time : Inport  Port=2
  AND : Logic  IconShape=distinctive  AllPortsSameDT=off  OutDataTypeStr=boolean
  Constant : Constant  Value=TM_Reset_Var
  Constant5 : Constant
  Equal : RelationalOperator  Operator===  OutDataTypeStr=boolean  RndMeth=Simplest
  Equal1 : RelationalOperator  Operator===  OutDataTypeStr=boolean  RndMeth=Simplest
  Reset Variables : Subsystem
  wires:
  AND/1 -> Reset Variables/Enable
  Equal/1 -> AND/2
  Equal1/1 -> AND/1
  basic cycle/1 -> Equal1/1
  Constant5/1 -> Equal1/2
  local time/1 -> Equal/1
  Constant/1 -> Equal/2

== system HANcoder_E407_GTSync_v5/HANcoder STM32 Target - E407-STM32 algorithm/Global Ticks Increment/CAN Management/Matrix Cycle Manager/COMP Task - Rx_Sync_Check ==
  note: BC 0 TW0
      | Sync Message
  note: Local Time still not updated
  basic_cycle : Inport
  local_time : Inport  Port=2
  new_CAN1_msg : Inport  Port=3
  new_CAN2_msg : Inport  Port=4
  Rx_msg_CAN1 : Inport  Port=5  OutDataTypeStr=Bus: msg_buffer_type
  Rx_msg_CAN2 : Inport  Port=6  OutDataTypeStr=Bus: msg_buffer_type
  AND : Logic  Inputs=3  IconShape=distinctive  AllPortsSameDT=off  OutDataTypeStr=boolean
  Constant : Constant  Value=TM_Check_Sync
  Constant1 : Constant  Value=TM_COMM_Sync
  Constant5 : Constant  Value=0
  Data Store Read : DataStoreRead  DataStoreName=Master_ID
  Data Store Read1 : DataStoreRead  DataStoreName=sync_processed
  Equal : RelationalOperator  Operator===  OutDataTypeStr=boolean  RndMeth=Simplest
  Equal1 : RelationalOperator  Operator===  OutDataTypeStr=boolean  RndMeth=Simplest
  NOT : Logic  Operator=NOT  IconShape=distinctive  AllPortsSameDT=off  OutDataTypeStr=boolean
  Process_Messages : Subsystem  Priority=20
  wires:
  new_CAN2_msg/1 -> Process_Messages/2(new_CAN2_msg)
  new_CAN1_msg/1 -> Process_Messages/1(new_CAN1_msg)
  basic_cycle/1 -> Process_Messages/7(expected_basic_cycle), Equal1/1
  local_time/1 -> Equal/1
  Equal/1 -> AND/2
  Equal1/1 -> AND/1
  Constant/1 -> Equal/2
  Constant5/1 -> Equal1/2
  AND/1 -> Process_Messages/Enable
  Rx_msg_CAN1/1 -> Process_Messages/3(Rx_msg_CAN1)
  Rx_msg_CAN2/1 -> Process_Messages/4(Rx_Msg_CAN2)
  Data Store Read/1 -> Process_Messages/5(expected_msg_header)
  Constant1/1 -> Process_Messages/6(expected_local_time)
  Data Store Read1/1 -> NOT/1
  NOT/1 -> AND/3

== system HANcoder_E407_GTSync_v5/HANcoder STM32 Target - E407-STM32 algorithm/Global Ticks Increment/CAN Management/Matrix Cycle Manager/COMP Task - Rx_Sync_Check - bc1 ==
  note: BC 1 TW0
      | Sync Message
  basic_cycle : Inport
  local_time : Inport  Port=2
  new_CAN1_msg : Inport  Port=3
  new_CAN2_msg : Inport  Port=4
  Rx_msg_CAN1 : Inport  Port=5  OutDataTypeStr=Bus: msg_buffer_type
  Rx_msg_CAN2 : Inport  Port=6  OutDataTypeStr=Bus: msg_buffer_type
  AND : Logic  IconShape=distinctive  AllPortsSameDT=off  OutDataTypeStr=boolean
  Constant : Constant  Value=TM_Check_Sync
  Constant1 : Constant  Value=TM_COMM_Sync
  Constant5 : Constant
  Data Store Read : DataStoreRead  DataStoreName=Master_ID
  Equal : RelationalOperator  Operator===  OutDataTypeStr=boolean  RndMeth=Simplest
  Equal1 : RelationalOperator  Operator===  OutDataTypeStr=boolean  RndMeth=Simplest
  Process_Messages : Subsystem
  wires:
  Constant1/1 -> Process_Messages/6(expected_local_time)
  Data Store Read/1 -> Process_Messages/5(expected_msg_header)
  Rx_msg_CAN2/1 -> Process_Messages/4(Rx_Msg_CAN2)
  Rx_msg_CAN1/1 -> Process_Messages/3(Rx_msg_CAN1)
  AND/1 -> Process_Messages/Enable
  Constant5/1 -> Equal1/2
  Constant/1 -> Equal/2
  Equal1/1 -> AND/1
  Equal/1 -> AND/2
  local_time/1 -> Equal/1
  basic_cycle/1 -> Process_Messages/7(expected_basic_cycle), Equal1/1
  new_CAN1_msg/1 -> Process_Messages/1(new_CAN1_msg)
  new_CAN2_msg/1 -> Process_Messages/2(new_CAN2_msg)

== system HANcoder_E407_GTSync_v5/HANcoder STM32 Target - E407-STM32 algorithm/Global Ticks Increment/CAN Management/Matrix Cycle Manager/COMP Task - Rx_Vote1_Check ==
  note: BC 0 TW0
      | Sync Message
  basic_cycle : Inport
  local_time : Inport  Port=2
  new_CAN1_msg : Inport  Port=3
  new_CAN2_msg : Inport  Port=4
  Rx_msg_CAN1 : Inport  Port=5  OutDataTypeStr=Bus: msg_buffer_type
  Rx_msg_CAN2 : Inport  Port=6  OutDataTypeStr=Bus: msg_buffer_type
  AND : Logic  IconShape=distinctive  AllPortsSameDT=off  OutDataTypeStr=boolean
  Constant : Constant  Value=TM_Check_Vote1
  Constant1 : Constant  Value=TM_COMM_Vote1
  Constant5 : Constant  Value=0
  Equal : RelationalOperator  Operator===  OutDataTypeStr=boolean  RndMeth=Simplest
  Equal1 : RelationalOperator  Operator===  OutDataTypeStr=boolean  RndMeth=Simplest
  Process_Messages1 : Subsystem
  wires:
  Constant1/1 -> Process_Messages1/5(expected_local_time)
  Rx_msg_CAN2/1 -> Process_Messages1/4(Rx_Msg_CAN2)
  Rx_msg_CAN1/1 -> Process_Messages1/3(Rx_msg_CAN1)
  AND/1 -> Process_Messages1/Enable
  Constant5/1 -> Equal1/2
  Constant/1 -> Equal/2
  Equal1/1 -> AND/1
  Equal/1 -> AND/2
  local_time/1 -> Equal/1
  basic_cycle/1 -> Process_Messages1/6(expected_basic_cycle), Equal1/1
  new_CAN1_msg/1 -> Process_Messages1/1(new_CAN1_msg)
  new_CAN2_msg/1 -> Process_Messages1/2(new_CAN2_msg)

== system HANcoder_E407_GTSync_v5/HANcoder STM32 Target - E407-STM32 algorithm/Global Ticks Increment/CAN Management/Matrix Cycle Manager/COMP Task - Rx_Vote2_Check ==
  note: BC 0 TW0
      | Sync Message
  basic_cycle : Inport
  local_time : Inport  Port=2
  new_CAN1_msg : Inport  Port=3
  new_CAN2_msg : Inport  Port=4
  Rx_msg_CAN1 : Inport  Port=5  OutDataTypeStr=Bus: msg_buffer_type
  Rx_msg_CAN2 : Inport  Port=6  OutDataTypeStr=Bus: msg_buffer_type
  AND : Logic  IconShape=distinctive  AllPortsSameDT=off  OutDataTypeStr=boolean
  Constant : Constant  Value=TM_Check_Vote2
  Constant1 : Constant  Value=TM_COMM_Vote2
  Constant5 : Constant  Value=0
  Equal : RelationalOperator  Operator===  OutDataTypeStr=boolean  RndMeth=Simplest
  Equal1 : RelationalOperator  Operator===  OutDataTypeStr=boolean  RndMeth=Simplest
  Process_Messages1 : Subsystem
  wires:
  new_CAN2_msg/1 -> Process_Messages1/2(new_CAN2_msg)
  new_CAN1_msg/1 -> Process_Messages1/1(new_CAN1_msg)
  basic_cycle/1 -> Process_Messages1/6(expected_basic_cycle), Equal1/1
  local_time/1 -> Equal/1
  Equal/1 -> AND/2
  Equal1/1 -> AND/1
  Constant/1 -> Equal/2
  Constant5/1 -> Equal1/2
  AND/1 -> Process_Messages1/Enable
  Rx_msg_CAN1/1 -> Process_Messages1/3(Rx_msg_CAN1)
  Rx_msg_CAN2/1 -> Process_Messages1/4(Rx_Msg_CAN2)
  Constant1/1 -> Process_Messages1/5(expected_local_time)

== system HANcoder_E407_GTSync_v5/HANcoder STM32 Target - E407-STM32 algorithm/Global Ticks Increment/CAN Management/Matrix Cycle Manager/COMP Task - Rx_Vote3_Check ==
  note: BC 0 TW0
      | Sync Message
  basic_cycle : Inport
  local_time : Inport  Port=2
  new_CAN1_msg : Inport  Port=3
  new_CAN2_msg : Inport  Port=4
  Rx_msg_CAN1 : Inport  Port=5  OutDataTypeStr=Bus: msg_buffer_type
  Rx_msg_CAN2 : Inport  Port=6  OutDataTypeStr=Bus: msg_buffer_type
  AND : Logic  IconShape=distinctive  AllPortsSameDT=off  OutDataTypeStr=boolean
  Constant : Constant  Value=TM_Check_Vote3
  Constant1 : Constant  Value=TM_COMM_Vote3
  Constant5 : Constant  Value=0
  Equal : RelationalOperator  Operator===  OutDataTypeStr=boolean  RndMeth=Simplest
  Equal1 : RelationalOperator  Operator===  OutDataTypeStr=boolean  RndMeth=Simplest
  Process_Messages1 : Subsystem
  wires:
  Constant1/1 -> Process_Messages1/5(expected_local_time)
  Rx_msg_CAN2/1 -> Process_Messages1/4(Rx_Msg_CAN2)
  Rx_msg_CAN1/1 -> Process_Messages1/3(Rx_msg_CAN1)
  AND/1 -> Process_Messages1/Enable
  Constant5/1 -> Equal1/2
  Constant/1 -> Equal/2
  Equal1/1 -> AND/1
  Equal/1 -> AND/2
  local_time/1 -> Equal/1
  basic_cycle/1 -> Process_Messages1/6(expected_basic_cycle), Equal1/1
  new_CAN1_msg/1 -> Process_Messages1/1(new_CAN1_msg)
  new_CAN2_msg/1 -> Process_Messages1/2(new_CAN2_msg)

== system HANcoder_E407_GTSync_v5/HANcoder STM32 Target - E407-STM32 algorithm/Global Ticks Increment/CAN Management/Matrix Cycle Manager/COMP Task - Update LT ==
  note: Local Time still not updated
  note: Sync Message received by Slave
  note: BC 0 TW1
      | Sync Message
  basic cycle : Inport
  local time : Inport  Port=2
  new_message : Inport  Port=3
  Rx_msg : Inport  Port=4
  AND : Logic  IconShape=distinctive  AllPortsSameDT=off  OutDataTypeStr=boolean
  AND1 : Logic  Inputs=3  IconShape=distinctive  AllPortsSameDT=off  OutDataTypeStr=boolean
  AND12 : Logic  IconShape=distinctive  AllPortsSameDT=off  OutDataTypeStr=boolean
  Bus Selector : BusSelector  OutputSignals=Msg_Header,Local_Time,Basic_Cycle
  Constant : Constant  Value=TM_Update_LT
  Constant4 : Constant  Value=Slave_Role
  Constant5 : Constant  Value=0
  Data Store Read : DataStoreRead  DataStoreName=sync_processed
  Data Store Read1 : DataStoreRead  DataStoreName=Role_ID
  Equal : RelationalOperator  Operator===  OutDataTypeStr=boolean  RndMeth=Simplest
  Equal1 : RelationalOperator  Operator===  OutDataTypeStr=boolean  RndMeth=Simplest
  Equal2 : RelationalOperator  Operator===  OutDataTypeStr=boolean  RndMeth=Simplest
  Local Time Update : Subsystem  Priority=20
  NOT : Logic  Operator=NOT  IconShape=distinctive  AllPortsSameDT=off  OutDataTypeStr=boolean
  Terminator : Terminator
  Terminator1 : Terminator
  Terminator2 : Terminator
  wires:
  Constant4/1 -> Equal2/2
  Data Store Read1/1 -> Equal2/1
  AND12/1 -> AND1/2
  Bus Selector/2 -> Terminator1/1  "<Local_Time>"
  Bus Selector/3 -> Terminator2/1  "<Basic_Cycle>"
  Equal2/1 -> AND12/2
  Bus Selector/1 -> Terminator/1  "<Msg_Header>"
  Equal1/1 -> AND/1
  basic cycle/1 -> Equal1/1
  Constant/1 -> Equal/2
  local time/1 -> Equal/1
  Equal/1 -> AND/2
  Constant5/1 -> Equal1/2
  AND1/1 -> Local Time Update/Enable
  AND/1 -> AND1/1
  new_message/1 -> AND12/1
  Rx_msg/1 -> Bus Selector/1
  Data Store Read/1 -> NOT/1
  NOT/1 -> AND1/3

== system HANcoder_E407_GTSync_v5/HANcoder STM32 Target - E407-STM32 algorithm/Global Ticks Increment/CAN Management/Matrix Cycle Manager/COMP Task - Update LT - bc1 ==
  note: BC 1 TW1
      | Sync Message
  note: Sync Message received by Slave
  note: Local Time still not updated
  basic cycle : Inport
  local time : Inport  Port=2
  new_message : Inport  Port=3
  Rx_msg : Inport  Port=4
  AND : Logic  IconShape=distinctive  AllPortsSameDT=off  OutDataTypeStr=boolean
  AND1 : Logic  Inputs=3  IconShape=distinctive  AllPortsSameDT=off  OutDataTypeStr=boolean
  AND12 : Logic  IconShape=distinctive  AllPortsSameDT=off  OutDataTypeStr=boolean
  Bus Selector : BusSelector  OutputSignals=Msg_Header,Local_Time,Basic_Cycle
  Constant : Constant  Value=TM_Update_LT
  Constant4 : Constant  Value=Slave_Role
  Constant5 : Constant
  Data Store Read : DataStoreRead  DataStoreName=sync_processed
  Data Store Read1 : DataStoreRead  DataStoreName=Role_ID
  Equal : RelationalOperator  Operator===  OutDataTypeStr=boolean  RndMeth=Simplest
  Equal1 : RelationalOperator  Operator===  OutDataTypeStr=boolean  RndMeth=Simplest
  Equal2 : RelationalOperator  Operator===  OutDataTypeStr=boolean  RndMeth=Simplest
  Local Time Update : Subsystem
  NOT : Logic  Operator=NOT  IconShape=distinctive  AllPortsSameDT=off  OutDataTypeStr=boolean
  Terminator : Terminator
  Terminator1 : Terminator
  Terminator2 : Terminator
  wires:
  Bus Selector/2 -> Terminator1/1  "<Local_Time>"
  Bus Selector/3 -> Terminator2/1  "<Basic_Cycle>"
  Bus Selector/1 -> Terminator/1  "<Msg_Header>"
  Equal1/1 -> AND/1
  basic cycle/1 -> Equal1/1
  Constant/1 -> Equal/2
  local time/1 -> Equal/1
  Equal/1 -> AND/2
  Constant5/1 -> Equal1/2
  AND1/1 -> Local Time Update/Enable
  AND/1 -> AND1/1
  Rx_msg/1 -> Bus Selector/1
  Data Store Read/1 -> NOT/1
  new_message/1 -> AND12/1
  Equal2/1 -> AND12/2
  AND12/1 -> AND1/2
  NOT/1 -> AND1/3
  Constant4/1 -> Equal2/2
  Data Store Read1/1 -> Equal2/1

== system HANcoder_E407_GTSync_v5/HANcoder STM32 Target - E407-STM32 algorithm/Global Ticks Increment/CAN Management/Matrix Cycle Manager/COMP Task - Vote Decision ==
  note: BC 0 TW2
      | Vote decision
  basic cycle : Inport
  local time : Inport  Port=2
  AND : Logic  IconShape=distinctive  AllPortsSameDT=off  OutDataTypeStr=boolean
  Constant : Constant  Value=TM_Vote_Dec
  Constant5 : Constant  Value=0
  Equal : RelationalOperator  Operator===  OutDataTypeStr=boolean  RndMeth=Simplest
  Equal1 : RelationalOperator  Operator===  OutDataTypeStr=boolean  RndMeth=Simplest
  Vote Decision : Subsystem  Priority=20
  wires:
  AND/1 -> Vote Decision/Enable
  Equal/1 -> AND/2
  Equal1/1 -> AND/1
  basic cycle/1 -> Equal1/1
  Constant5/1 -> Equal1/2
  local time/1 -> Equal/1
  Constant/1 -> Equal/2

== system HANcoder_E407_GTSync_v5/HANcoder STM32 Target - E407-STM32 algorithm/Global Ticks Increment/CAN Management/Matrix Cycle Manager/COMP Task - Vote1 Count ==
  note: BC 0 TW4
      | Vote 1 Message
  note: Vote 1 received by
      | other boards
  basic cycle : Inport
  local time : Inport  Port=2
  new_message : Inport  Port=3
  Rx_msg : Inport  Port=4
  AND : Logic  IconShape=distinctive  AllPortsSameDT=off  OutDataTypeStr=boolean
  AND1 : Logic  IconShape=distinctive  AllPortsSameDT=off  OutDataTypeStr=boolean
  AND12 : Logic  IconShape=distinctive  AllPortsSameDT=off  OutDataTypeStr=boolean
  Bus Selector : BusSelector  OutputSignals=Msg_Header,Local_Time,Basic_Cycle
  Constant : Constant  Value=TM_Count_Vote1
  Constant4 : Constant
  Constant5 : Constant  Value=0
  Data Store Read1 : DataStoreRead  DataStoreName=Board_ID
  Equal : RelationalOperator  Operator===  OutDataTypeStr=boolean  RndMeth=Simplest
  Equal1 : RelationalOperator  Operator===  OutDataTypeStr=boolean  RndMeth=Simplest
  Equal2 : RelationalOperator  Operator=~=  OutDataTypeStr=boolean  RndMeth=Simplest
  Terminator1 : Terminator
  Terminator2 : Terminator
  Vote Count 1 : Subsystem
  wires:
  AND/1 -> AND1/1
  AND1/1 -> Vote Count 1/Enable
  Constant5/1 -> Equal1/2
  Equal/1 -> AND/2
  local time/1 -> Equal/1
  Constant/1 -> Equal/2
  basic cycle/1 -> Equal1/1
  Equal1/1 -> AND/1
  Equal2/1 -> AND12/2
  AND12/1 -> AND1/2
  Data Store Read1/1 -> Equal2/1
  Constant4/1 -> Equal2/2
  new_message/1 -> AND12/1
  Bus Selector/2 -> Terminator2/1  "<Local_Time>"
  Bus Selector/1 -> Vote Count 1/1(Msg Header)  "<Msg_Header>"
  Bus Selector/3 -> Terminator1/1  "<Basic_Cycle>"
  Rx_msg/1 -> Bus Selector/1

== system HANcoder_E407_GTSync_v5/HANcoder STM32 Target - E407-STM32 algorithm/Global Ticks Increment/CAN Management/Matrix Cycle Manager/COMP Task - Vote2 Count ==
  note: Vote 2 received by
      | other boards
  note: BC 0 TW6
      | Vote 1 Message
  basic cycle : Inport
  local time : Inport  Port=2
  new_message : Inport  Port=3
  Rx_msg : Inport  Port=4
  AND : Logic  IconShape=distinctive  AllPortsSameDT=off  OutDataTypeStr=boolean
  AND1 : Logic  IconShape=distinctive  AllPortsSameDT=off  OutDataTypeStr=boolean
  AND12 : Logic  IconShape=distinctive  AllPortsSameDT=off  OutDataTypeStr=boolean
  Bus Selector : BusSelector  OutputSignals=Msg_Header,Local_Time,Basic_Cycle
  Constant : Constant  Value=TM_Count_Vote2
  Constant4 : Constant  Value=2
  Constant5 : Constant  Value=0
  Data Store Read1 : DataStoreRead  DataStoreName=Board_ID
  Equal : RelationalOperator  Operator===  OutDataTypeStr=boolean  RndMeth=Simplest
  Equal1 : RelationalOperator  Operator===  OutDataTypeStr=boolean  RndMeth=Simplest
  Equal2 : RelationalOperator  Operator=~=  OutDataTypeStr=boolean  RndMeth=Simplest
  Terminator1 : Terminator
  Terminator2 : Terminator
  Vote Count 2 : Subsystem
  wires:
  Constant4/1 -> Equal2/2
  Data Store Read1/1 -> Equal2/1
  AND12/1 -> AND1/2
  Equal2/1 -> AND12/2
  Equal1/1 -> AND/1
  basic cycle/1 -> Equal1/1
  Constant/1 -> Equal/2
  local time/1 -> Equal/1
  Equal/1 -> AND/2
  Constant5/1 -> Equal1/2
  AND1/1 -> Vote Count 2/Enable
  AND/1 -> AND1/1
  new_message/1 -> AND12/1
  Bus Selector/3 -> Terminator1/1  "<Basic_Cycle>"
  Bus Selector/1 -> Vote Count 2/1(Msg Header)  "<Msg_Header>"
  Bus Selector/2 -> Terminator2/1  "<Local_Time>"
  Rx_msg/1 -> Bus Selector/1

== system HANcoder_E407_GTSync_v5/HANcoder STM32 Target - E407-STM32 algorithm/Global Ticks Increment/CAN Management/Matrix Cycle Manager/COMP Task - Vote3 Count ==
  note: BC 0 TW8
      | Vote 3 Message
  note: Vote 3 received by
      | other boards
  basic cycle : Inport
  local time : Inport  Port=2
  new_message : Inport  Port=3
  Rx_msg : Inport  Port=4
  AND : Logic  IconShape=distinctive  AllPortsSameDT=off  OutDataTypeStr=boolean
  AND1 : Logic  IconShape=distinctive  AllPortsSameDT=off  OutDataTypeStr=boolean
  AND12 : Logic  IconShape=distinctive  AllPortsSameDT=off  OutDataTypeStr=boolean
  Bus Selector : BusSelector  OutputSignals=Msg_Header,Local_Time,Basic_Cycle
  Constant : Constant  Value=TM_Count_Vote3
  Constant4 : Constant  Value=3
  Constant5 : Constant  Value=0
  Data Store Read1 : DataStoreRead  DataStoreName=Board_ID
  Equal : RelationalOperator  Operator===  OutDataTypeStr=boolean  RndMeth=Simplest
  Equal1 : RelationalOperator  Operator===  OutDataTypeStr=boolean  RndMeth=Simplest
  Equal2 : RelationalOperator  Operator=~=  OutDataTypeStr=boolean  RndMeth=Simplest
  Terminator1 : Terminator
  Terminator2 : Terminator
  Vote Count 3 : Subsystem
  wires:
  AND/1 -> AND1/1
  AND1/1 -> Vote Count 3/Enable
  Constant5/1 -> Equal1/2
  Equal/1 -> AND/2
  local time/1 -> Equal/1
  Constant/1 -> Equal/2
  basic cycle/1 -> Equal1/1
  Equal1/1 -> AND/1
  Equal2/1 -> AND12/2
  AND12/1 -> AND1/2
  Data Store Read1/1 -> Equal2/1
  Constant4/1 -> Equal2/2
  new_message/1 -> AND12/1
  Bus Selector/1 -> Vote Count 3/1(Msg Header)  "<Msg_Header>"
  Rx_msg/1 -> Bus Selector/1
  Bus Selector/3 -> Terminator1/1  "<Basic_Cycle>"
  Bus Selector/2 -> Terminator2/1  "<Local_Time>"

== system HANcoder_E407_GTSync_v5/HANcoder STM32 Target - E407-STM32 algorithm/Global Ticks Increment/CAN Management/Matrix Cycle Manager/LT_Update Desync_Positive ==
  note: Local Time Update with Positive Desync
      | This subsystem is only activated if we have to update
      | the local time with a positive desyn. This is activated
      | at the end of the current Computational Task, so the
      | Local Time is updated until the tick before the next
      | Computational Task in the basic cycle. This way we
      | avoid missing tasks, as would happend when updating
      | the Local Time too quickly into the future.
  Local Time : Inport
  Enable : EnablePort
  Desync update calculation : Subsystem
  Local Time Update with Positive Desync : Subsystem  TreatAsAtomicUnit=on
  Subsystem : Subsystem
  wires:
  Local Time/1 -> Subsystem/1(Local Time), Desync update calculation/1(Local Time)
  Desync update calculation/1(Update Desync Value) -> Local Time Update with Positive Desync/1(Ticks until next COMP)
  Subsystem/1(No TM condition) -> Local Time Update with Positive Desync/Enable
